simulink model "Copy_of_DEES_2d"  (R2019a)
settings: Solver=VariableStepAuto  StartTime=0.0  StopTime=1000  RelTol=1e-3
settings Model: Creator=Bhavya  LastModifiedBy=Bhavya

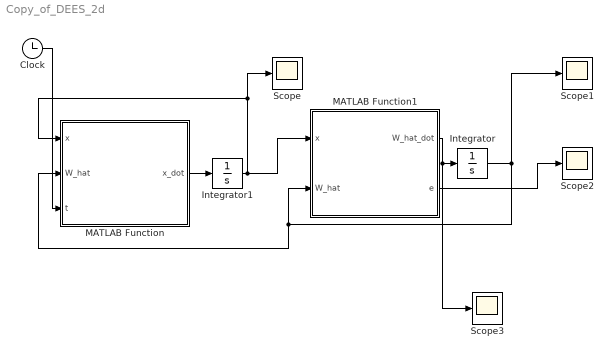
== system Copy_of_DEES_2d ==
  Clock : Clock
  Integrator : Integrator  InitialCondition=[0;0;0;0;0;0]
  Integrator1 : Integrator  InitialCondition=[3;4]
  MATLAB Function : MATLAB Function  TreatAsAtomicUnit=on
  MATLAB Function1 : MATLAB Function  TreatAsAtomicUnit=on
  Scope{,1..3} (4 alike) : Scope
  wires:
  MATLAB Function/1(x_dot) -> Integrator1/1
  MATLAB Function1/1(W_hat_dot) -> Scope3/1, Integrator/1
  Integrator1/1 -> Scope/1, MATLAB Function/1(x), MATLAB Function1/1(x)
  Integrator/1 -> MATLAB Function/2(W_hat), MATLAB Function1/2(W_hat), Scope1/1
  Clock/1 -> MATLAB Function/3(t)
  MATLAB Function1/2(e) -> Scope2/1

== matlab function Copy_of_DEES_2d/MATLAB Function1 ==
  data: x input; W_hat_dot output; W_hat input; e output
function [W_hat_dot,e]= Estimator(x,W_hat)
x1=x(1,1);
x2=x(2,1);
phi=[x1^2;x2^2;x1*x2;x1;x2;1];

f_hat=W_hat'*phi;
W_star=[1;1;0;-4;-4;8];
alpha=1;
f_data=W_star'*phi;

e=f_hat-f_data;

W_hat_dot=(-alpha*e)*phi/(1+phi'*phi)^2;

== matlab function Copy_of_DEES_2d/MATLAB Function ==
  data: x input; x_dot output; W_hat input; t input
% function r=P_k(x)
%     mini =0;
%     for i=1:0.5:10
%         if abs(i-x)<abs(mini-x)
%             mini=i;
%         end
%     end
%     r=mini;
% end

function x_dot = Dynamics(x,W_hat,t)
x1=x(1,1);
x2=x(2,1);
phi=[x1^2;x2^2;x1*x2;x1;x2;1];
%jac=@(y)jacobian(phi(y));
jac_2=[2*x1 0;0 2*x2;x2 x1;1 0;0 1;0 0];
%x_dot=-x+P_k(x-W_hat'*jac_2(x));

x_dot=0.1*(-(W_hat'*jac_2)'+exp(-0.0000001*t)*[sin(pi*t)+cos(2*t)+sin(sqrt(2)*t)+cos(3*t);sin(2*t)+cos(sqrt(3)*t)+sin(3*(pi/4)*t)+cos(8*t)]);
% if(t<150)
%     del=1*[sin(pi*t)+cos(2*pi*t)+sin(sqrt(2)*t)+cos(4*pi*t);sin(2*t)+cos(sqrt(3)*t)+sin(6*t)+cos(8*t)];
% else
%     del=1*exp(-0.00001*(t-150))*[sin(pi*t)+cos(2*pi*t)+sin(sqrt(2)*t)+cos(4*pi*t);sin(2*t)+cos(sqrt(3)*t)+sin(6*t)+cos(8*t)];
% end
% x_dot=0.1*(-(W_hat'*jac_2)'+del);
end
